simulink model "Sensor_Failure_Detection"  (R2023b)
settings: Solver=FixedStepDiscrete  StartTime=0.0  StopTime=10.0  FixedStep=.1  RelTol=1e-3
settings Model: Creator=MOHAMED  LastModifiedBy=MOHAMED

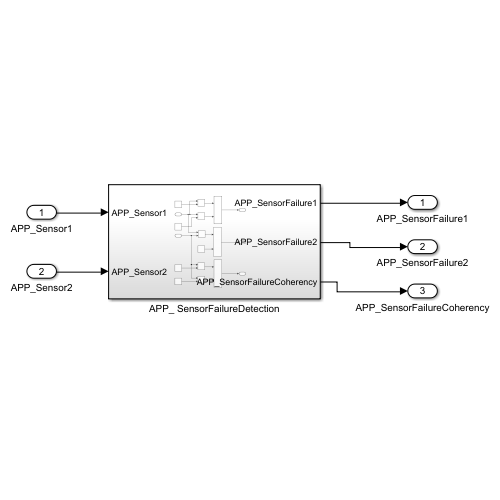
[thumbnail: Simulink's stored preview of the top-level diagram]
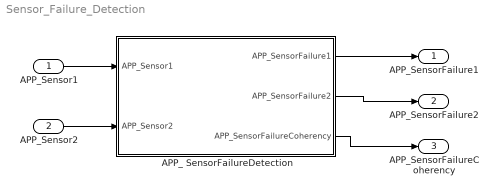
== system Sensor_Failure_Detection ==
  APP_Sensor1 : Inport
  APP_Sensor2 : Inport  Port=2
  APP_ SensorFailureDetection : Subsystem
  APP_SensorFailure1 : Outport
  APP_SensorFailure2 : Outport  Port=2
  APP_SensorFailureCoherency : Outport  Port=3
  wires:
  APP_ SensorFailureDetection/1(APP_SensorFailure1) -> APP_SensorFailure1/1
  APP_Sensor1/1 -> APP_ SensorFailureDetection/1(APP_Sensor1)
  APP_Sensor2/1 -> APP_ SensorFailureDetection/2(APP_Sensor2)
  APP_ SensorFailureDetection/3(APP_SensorFailureCoherency) -> APP_SensorFailureCoherency/1
  APP_ SensorFailureDetection/2(APP_SensorFailure2) -> APP_SensorFailure2/1

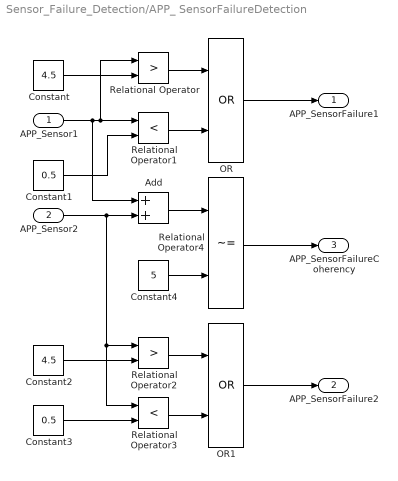
== system Sensor_Failure_Detection/APP_ SensorFailureDetection ==
  APP_Sensor1 : Inport
  APP_Sensor2 : Inport  Port=2
  Add : Sum
  Constant : Constant  Value=4.5
  Constant1 : Constant  Value=0.5
  Constant2 : Constant  Value=4.5
  Constant3 : Constant  Value=0.5
  Constant4 : Constant  Value=5
  OR : Logic  Operator=OR  AllPortsSameDT=off  OutDataTypeStr=boolean
  OR1 : Logic  Operator=OR  AllPortsSameDT=off  OutDataTypeStr=boolean
  Relational Operator : RelationalOperator  Operator=>  OutDataTypeStr=boolean  RndMeth=Simplest  InputSameDT=off
  Relational Operator1 : RelationalOperator  Operator=<  OutDataTypeStr=boolean  RndMeth=Simplest  InputSameDT=off
  Relational Operator2 : RelationalOperator  Operator=>  OutDataTypeStr=boolean  RndMeth=Simplest  InputSameDT=off
  Relational Operator3 : RelationalOperator  Operator=<  OutDataTypeStr=boolean  RndMeth=Simplest  InputSameDT=off
  Relational Operator4 : RelationalOperator  Operator=~=  OutDataTypeStr=boolean  RndMeth=Simplest  InputSameDT=off
  APP_SensorFailure1 : Outport
  APP_SensorFailure2 : Outport  Port=2
  APP_SensorFailureCoherency : Outport  Port=3
  wires:
  Relational Operator/1 -> OR/1
  Constant1/1 -> Relational Operator1/2
  Constant/1 -> Relational Operator/2
  APP_Sensor1/1 -> Relational Operator1/1, Relational Operator/1, Add/1
  APP_Sensor2/1 -> Relational Operator3/1, Relational Operator2/1, Add/2
  Constant3/1 -> Relational Operator3/2
  Relational Operator3/1 -> OR1/2
  Constant2/1 -> Relational Operator2/2
  OR/1 -> APP_SensorFailure1/1
  Relational Operator1/1 -> OR/2
  Add/1 -> Relational Operator4/1
  Relational Operator4/1 -> APP_SensorFailureCoherency/1
  Constant4/1 -> Relational Operator4/2
  Relational Operator2/1 -> OR1/1
  OR1/1 -> APP_SensorFailure2/1
